simulink model "Part1_windturbine"  (R2022b)
settings: Solver=FixedStepAuto  StartTime=0.0  StopTime=30  FixedStep=0.01  RelTol=1e-3
libraries: simulink x3
settings Model: Creator=lenovo  LastModifiedBy=mingreico

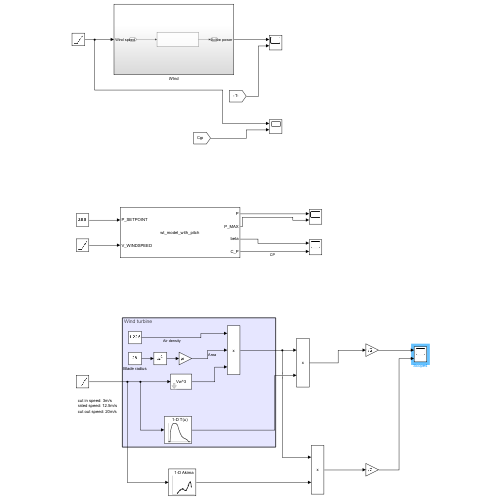
[thumbnail: Simulink's stored preview of the top-level diagram]
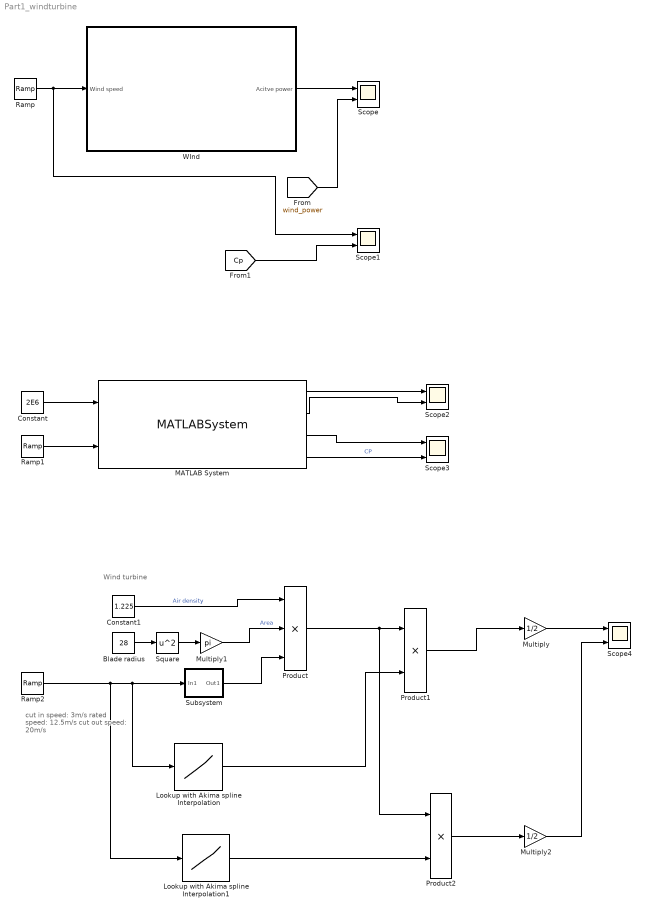
== system Part1_windturbine ==
  note: cut in speed: 3m/s
      | rated speed: 12.5m/s
      | cut out speed: 20m/s
  note: Wind turbine
  Blade radius : Constant  Value=28
  Constant : Constant  Value=2E6
  Constant1 : Constant  Value=1.225
  Lookup with Akima spline Interpolation : Lookup_n-D  NumberOfTableDimensions=1  BreakpointsForDimension1=[0;1;2;3;4;5;6;7;8;9;10;11;12;13;14;15;16;17;18;19;20;21;22;23;24;25;26;27;28]  Table=[0;0;0;0.228;0.322;0.38;0.408;0.413;0.418;0.419;0.419;0.401;0.378;0.305;0.244;0.199;0.164;0.136;0.115;0.098;0.084;0.072;0.063;0.055;0.048;0.042;0;0;0]  InternalRulePriority=Speed  OutDataTypeStr=double  RndMeth=Simplest
  Lookup with Akima spline Interpolation1 : Lookup_n-D  NumberOfTableDimensions=1  BreakpointsForDimension1=[0;1;2;3;4;5;6;7;8;9;10;11;12;13;14;15;16;17;18;19;20;21;22;23;24;25;26;27;28]  Table=[0;0;0;0.228;0.322;0.38;0.408;0.413;0.418;0.419;0.419;0.401;0.378;0.305;0.244;0.199;0.164;0.136;0.115;0.098;0.084;0.072;0.063;0.055;0.048;0.042;0;0;0]  InterpMethod=Akima spline  InternalRulePriority=Speed  OutDataTypeStr=double  RndMeth=Simplest
  MATLAB System : MATLABSystem  System=wt_model_with_pitch  turbine_Pinst=2e6  turbine_dynamicsTimeConstant=10  inertia_dynamicsTimeConstant=3  pitch_inertia_dynamicsPitchRate=2  Ts=0.01  SimulateUsing=Code generation
      mask Type: wt_model_with_pitch
      mask Display:
      | disp('wt_model_with_pitch');
      | port_label('input',1,'P_SETPOINT');
      | port_label('input',2,'V_WINDSPEED');
      | port_label('output',1,'P');
      | port_label('output',2,'P_MAX');
      | port_label('output',3,'beta');
      | port_label('output',4,'C_P');
  Multiply : Gain  Gain=1/2
  Multiply1 : Gain  Gain=pi
  Multiply2 : Gain  Gain=1/2
  Product : Product  Inputs=3
  Product1 : Product
  Product2 : Product
  Ramp : simulink/Sources/Ramp  slope=1  start=0  InitialOutput=0.0000001
  Ramp1 : simulink/Sources/Ramp  slope=1  start=0  InitialOutput=0.0000001
  Ramp2 : simulink/Sources/Ramp  slope=1  start=0  InitialOutput=0
  Scope{,1..4} (5 alike) : Scope  NumInputPorts=2
  Square : Math  Operator=square
  Subsystem : Subsystem
      mask Display: disp('Vw^3');
  WInd : Subsystem
  wires:
  WInd/1(Acitve power) -> Scope/1
  Ramp/1 -> Scope1/1, WInd/1(Wind speed)
  [Cp] -> Scope1/2
  [wind_power] -> Scope/2
  Ramp1/1 -> MATLAB System/2
  MATLAB System/1 -> Scope2/1
  MATLAB System/2 -> Scope2/2
  MATLAB System/4 -> Scope3/2  "CP"
  MATLAB System/3 -> Scope3/1
  Constant/1 -> MATLAB System/1
  Multiply1/1 -> Product/2  "Area"
  Square/1 -> Multiply1/1
  Constant1/1 -> Product/1  "Air density"
  Multiply/1 -> Scope4/1
  Blade radius/1 -> Square/1
  Ramp2/1 -> Lookup with Akima spline Interpolation1/1, Lookup with Akima spline Interpolation/1, Subsystem/1(In1)
  Subsystem/1(Out1) -> Product/3
  Product/1 -> Product2/1, Product1/1
  Lookup with Akima spline Interpolation/1 -> Product1/2
  Lookup with Akima spline Interpolation1/1 -> Product2/2
  Product1/1 -> Multiply/1
  Product2/1 -> Multiply2/1
  Multiply2/1 -> Scope4/2

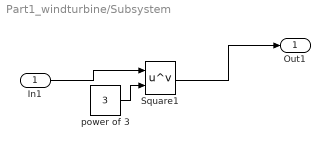
== system Part1_windturbine/Subsystem ==
  In1 : Inport
  Square1 : Math  Operator=pow
  power of 3 : Constant  Value=3
  Out1 : Outport
  wires:
  power of 3/1 -> Square1/2
  Square1/1 -> Out1/1
  In1/1 -> Square1/1

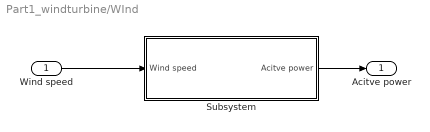
== system Part1_windturbine/WInd ==
  Wind speed : Inport
  Subsystem : Subsystem
  Acitve power : Outport
  wires:
  Subsystem/1(Acitve power) -> Acitve power/1
  Wind speed/1 -> Subsystem/1(Wind speed)

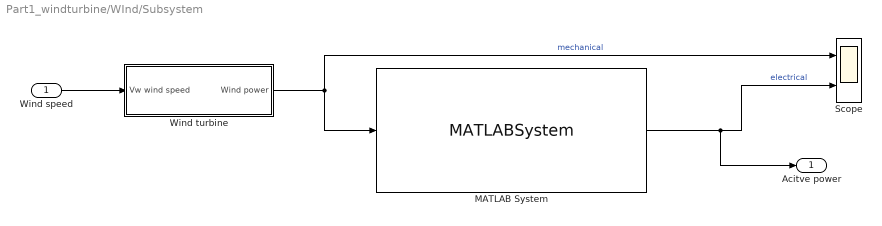
== system Part1_windturbine/WInd/Subsystem ==
  Wind speed : Inport
  MATLAB System : MATLABSystem  System=windturbine_pitch_control  turbine_Pinst=1e6  turbine_dynamicsTimeConstant=5  inertia_dynamicsTimeConstant=3  Ts=0.01  SimulateUsing=Code generation
      mask Type: windturbine_pitch_control
      mask Display:
      | disp('windturbine_pitch_control');
      | port_label('input',1,'P_mechanic');
      | port_label('output',1,'P');
  Scope : Scope  NumInputPorts=2
  Wind turbine : Subsystem  mask{C1=0.5, C2=116, C3=0.4, C4=0, C5=5, C6=21, theta=0, W=1.57, R=40}
      mask prompts: C1 "coefficients C1"; C2 "coefficients C2"; C3 "coefficients C3"; C4 "coefficients C4"; C5 "coefficients C5"; C6 "coefficients C6"; theta "pitch angle"; W "angular velocity of rotor"; R "Blade Radius"
      mask DialogControl Container4 Prompt: Cp power coefficient
      mask DialogControl Container3 Prompt: Blade parameter
  Acitve power : Outport
  wires:
  Wind speed/1 -> Wind turbine/1(Vw wind speed)
  Wind turbine/1(Wind power) -> MATLAB System/1, Scope/1  "mechanical"
  MATLAB System/1 -> Acitve power/1, Scope/2  "electrical"

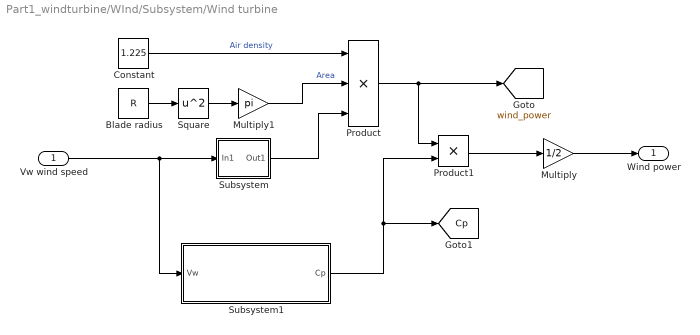
== system Part1_windturbine/WInd/Subsystem/Wind turbine ==
  Vw wind speed : Inport
  Blade radius : Constant  Value=R
  Constant : Constant  Value=1.225
  Multiply : Gain  Gain=1/2
  Multiply1 : Gain  Gain=pi
  Product : Product  Inputs=3
  Product1 : Product
  Square : Math  Operator=square
  Subsystem : Subsystem
      mask Display: disp('Vw^3');
  Subsystem1 : Subsystem
  Wind power : Outport
  tag scope: Cp=global, wind_power=global
  wires:
  Multiply/1 -> Wind power/1
  Constant/1 -> Product/1  "Air density"
  Blade radius/1 -> Square/1
  Square/1 -> Multiply1/1
  Multiply1/1 -> Product/2  "Area"
  Vw wind speed/1 -> Subsystem1/1(Vw), Subsystem/1(In1)
  Subsystem/1(Out1) -> Product/3
  Product1/1 -> Multiply/1
  Subsystem1/1(Cp) -> [Cp], Product1/2
  Product/1 -> [wind_power], Product1/1

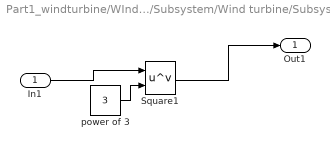
== system Part1_windturbine/WInd/Subsystem/Wind turbine/Subsystem ==
  In1 : Inport
  Square1 : Math  Operator=pow
  power of 3 : Constant  Value=3
  Out1 : Outport
  wires:
  power of 3/1 -> Square1/2
  Square1/1 -> Out1/1
  In1/1 -> Square1/1

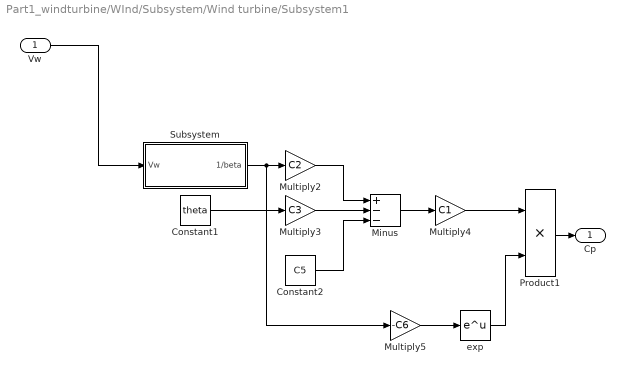
== system Part1_windturbine/WInd/Subsystem/Wind turbine/Subsystem1 ==
  Vw : Inport
  Constant1 : Constant  Value=theta
  Constant2 : Constant  Value=C5
  Minus : Sum  Inputs=+--
  Multiply2 : Gain  Gain=C2
  Multiply3 : Gain  Gain=C3
  Multiply4 : Gain  Gain=C1
  Multiply5 : Gain  Gain=-C6
  Product1 : Product
  Subsystem : Subsystem
  exp : Math
  Cp : Outport
  wires:
  Constant1/1 -> Multiply3/1
  Constant2/1 -> Minus/3
  Vw/1 -> Subsystem/1(Vw)
  Multiply2/1 -> Minus/1
  Minus/1 -> Multiply4/1
  Multiply4/1 -> Product1/1
  Subsystem/1(1/beta) -> Multiply5/1, Multiply2/1
  Multiply3/1 -> Minus/2
  exp/1 -> Product1/2
  Multiply5/1 -> exp/1
  Product1/1 -> Cp/1

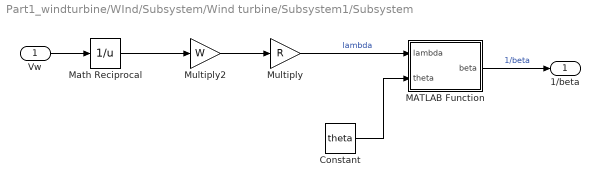
== system Part1_windturbine/WInd/Subsystem/Wind turbine/Subsystem1/Subsystem ==
  Vw : Inport
  Constant : Constant  Value=theta
  MATLAB Function : MATLAB Function  TreatAsAtomicUnit=on
  Math Reciprocal : Math  Operator=reciprocal  SignedPower=on
  Multiply : Gain  Gain=R
  Multiply2 : Gain  Gain=W
  1/beta : Outport
  wires:
  Multiply/1 -> MATLAB Function/1(lambda)  "lambda"
  Constant/1 -> MATLAB Function/2(theta)
  MATLAB Function/1(beta) -> 1/beta/1  "1/beta"
  Vw/1 -> Math Reciprocal/1
  Multiply2/1 -> Multiply/1
  Math Reciprocal/1 -> Multiply2/1

== matlab function Part1_windturbine/WInd/Subsystem/Wind turbine/Subsystem1/Subsystem/MATLAB Function ==
  data: lambda input; beta output; theta input
function beta  = fcn(lambda,theta)
%#codegen
    beta= 1/(lambda+0.08*theta)-0.035/(1+theta^3);
end
